simulink model "Cruise_Model_RebuildControl"  (R2024a)
settings: Solver=ode23t  StartTime=0.0  StopTime=20  RelTol=1e-3
values from neighbouring files (symbols this model uses):
  coefficients =     [UAM2.mat]    (also in VX4_cur.mat; VX4data.mat; alexisignoringme11UAM2.mat; alexisignoringme12.mat)
  K = lqr(sys, Q, R)    [QRerr.m]    (also in QRerr_p.m; alexisignoringme4.mat = [-2.3054870934e-16 -3.29424508508e-08 -2.01640092228e-07 -0.; alexisignoringme5.mat = [-2.3054870934e-16 -3.29424508508e-08 -2.01640092228e-07 -0.; alexisignoringme6.mat = [-2.3054870934e-16 -3.29424508508e-08 -2.01640092228e-07 -0.)
  mission =     [alexisignoringme.mat]    (also in alexisignoringme11UAM2.mat; alexisignoringme12.mat; alexisignoringme13.mat; alexisignoringme14.mat)
  q = 0.5*1.225*airflow.U^2    [VLMV3.m]    (also in VLMV3_modified.m = 0.5*1.225*airflow.U^2*Sref)
  referenceGeo =     [VX4data.mat]    (also in alexisignoringme.mat; alexisignoringme11UAM2.mat; alexisignoringme12.mat; alexisignoringme13.mat)
  Ue = U(:,idx(2)+1)    [QRerr.m]    (also in QRerr_LQI.m; QRerr_p.m; alexisignoringme4.mat = [0.01662518914 6.61806403433e-08 9.21309449136e-07 1460.2523; alexisignoringme5.mat = [0 0 0 0 0 -1471.90874183 1.06985703496e-06 -4.11944256484e-)
  X = [0.00351660116596 0 -9.99999602467 0 0 0 2.75026701025e-08 -4.1982332666e-06 -1.5333765693e-08 0.000503097278932 0 -6.54626389426e-11 ... (630 elements, 9x5x14)]    [alexisignoringme.mat]    (also in alexisignoringme12.mat = [0.000256495736971 0 -9.99999647184 0 0 0 0 -3.73764411116e-; alexisignoringme13.mat = [0.00833666803911 0 -10.0000021435 0 0 0 0 7.14203458163e-06; alexisignoringme14.mat = [0.00833666803911 0 -10.0000021435 0 0 0 0 7.14203458163e-06; alexisignoringme4.mat = [0.00351658839646 0 -9.99999599468 0 0 0 2.7327442949e-09 -4)
  Xes = X(:,idx(2))    [QRerr.m]    (also in QRerr_LQI.m; QRerr_p.m; alexisignoringme4.mat = [0.00351658839646 0 -9.99999599468 0 0 0 2.7327442949e-09 -4; alexisignoringme5.mat = [0 0 -1.11199998303 0 0 0 -1.38069247376e-09 1.48137256273e-)
undefined symbols (not defined in the file or in its folder): F, Light, MIL, VX4
libraries: slpidlib x14, aerolibwind2 x8, aerolibatmos2 x4, shared6dof x1
(part 1 of 3)
settings Model: Creator=Jem  LastModifiedBy=Jem
settings OptimizationCC: ReuseModelBlockBuffer=off
settings RTWCC: GPUComputeCapability=3.5

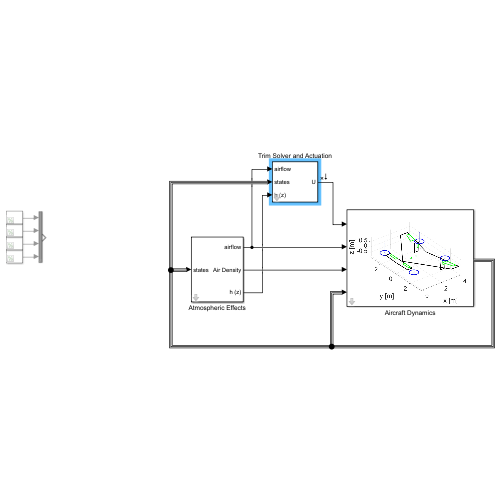
[thumbnail: Simulink's stored preview of the top-level diagram]
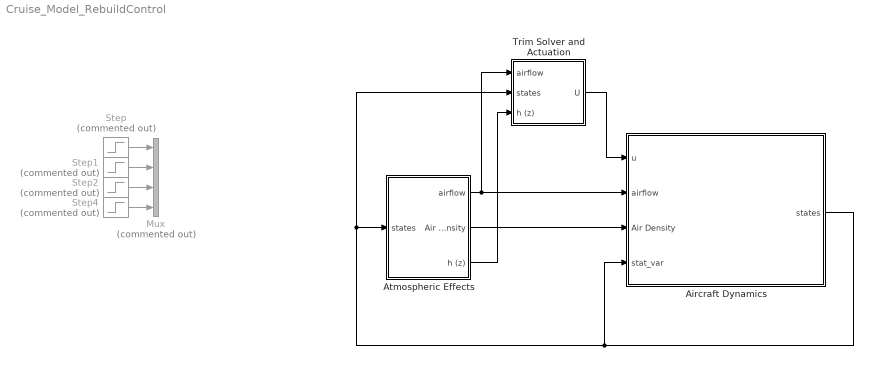
== system Cruise_Model_RebuildControl ==
  Aircraft Dynamics : Subsystem  mask{stabDeriv_local=0, config=VX4, refGeo=VX4.refGeo, mesh=[], stabDeriv=coefficients, I=[107 0 0.6971;0 93 0;0.6971 0 196], ac=[2.04 0 0], cg=[1.51 0 0], m=150, uvw=Xes(1:3), lmn=Xes(7:9), pqr=Xes(4:6), xyz_e=[0 0 0], CD0=0.038, CL0=0.3, Cm0=-0.02, CDa=0.1194, CLa=3.9492, CYa=0, CDb=0, CLb=0, CYb=-0.1997, Clla=0, Cma=-0.3679, Cna=0, Cllb=-0.1796, Cmb=0, Cnb=0.0421, CDn=[0 0 0], CLn=[0.1977 0 0], CYn=[0 0.01532 0.0984], Clln=[0 0.1366 -0.0126], Cmn=[0.2941 0 0], Cnn=[0 -0.0107 -0.03229], CYp=-0.1211, CYr=0.2494, CLq=4.7784, Clp=-0.3291, Clr=0.1134, Cmq=-2.4803, Cnp=0.01634, Cnr=-0.0387, kt=[3.13e-05;3.13e-05;3.13e-05;3.13e-05], kb=[7.5e-07;7.5e-07;7.5e-07;7.5e-07], Tinit=[0 0 0 0], xyz_tr=[3.7 1.75 0;3.7 -1.75 0;0.25 -2 0;0.25 2 0], anginit=[0 0 0;0 0 0;0 0 0;0 0 0], max_def_tr=[1 -1;1 -1;1 -1;1 -1], dir=[1;-1;1;-1]}
      mask prompts: config "Configuration (object)"; refGeo "Reference Geometry (struct)"; mesh "Mesh (struct)"; stabDeriv "Stability Derivatives (struct)"; I "Inertia Tensor"; ac "Aerodynamic Centre [x y z]_ref"; cg "Centre of Gravity [x y z]_ref"; m "Mass [kg]"; uvw "[u, v, w]"; lmn "[roll, pitch, yaw]"; pqr "[p, q, r]"; xyz_e "[Xe, Ye, Ze]"; CDa "CD_a"; CLa "CL_a"; CYa "CY_a"; CDb "CD_b"; CLb "CL_b"; CYb "CY_b"; Clla "Cl_a"; Cma "Cm_a"; Cna "Cn_a"; Cllb "Cl_b"; Cmb "Cm_b"; Cnb "Cn_b"; CDn "CD_n"; CLn "CL_n"; CYn "CY_n"; Clln "Cl_n"; Cmn "Cm_n"; Cnn "Cn_n"; Tinit "Initial Thrust [kN]"; xyz_tr "XYZ_b Pos [m]"; anginit "Initial ang_b [rad]"; max_def_tr "Max [+ve -ve] Deflection (from baseline) [rad]"; dir "Rot. Dir. ([1:Clockwise, -1:Anticlockwise])"
      mask Callback config:
      | config = get_param(gcb, 'config');
      |     m = Simulink.Mask.get(gcb);
      | 
      |     if config ~= "[]"
      |     try
      |         I = evalin('base',[config '.I']);
      |         I_mask = m.getParameter('I');
      |         I_mask.Value = mat2str(I);
      | 
      |         CoL = evalin('base', [config '.CoL']);
      |         CoL_mask = m.getParameter('ac');
      |         CoL_mask.Value = mat2str(CoL);
      | 
      |         CG = evalin('base', [config '.CG']);
      |         CG_mask = m.getParameter('cg');
      |         CG_mask.Value = mat2str(CG);
      | 
      |         Cd0 = evalin('base', [config '.Cd0']);
      |         Cd0_mask = m.getParameter('CD0');
      |         Cd0_mask.Value = mat2str(Cd0);
      | 
      |         mass = evalin('base', [config '.m']);
      |         mass_mask = m.getParameter('m');
      |         mass_mask.Value = mat2str(mass);
      | 
      |         thrustObjs = evalin('base', [config '.thrust']);
      |         xyz_tr = m.getParameter('xyz_tr');
      |         anginit = m.getParameter('anginit');
      |         max_def_tr = m.getParameter('max_def_tr');
      |         Tinit = m.getParameter('Tinit');
      | 
      |         kb = m.getParameter('kb');
      |         kt = m.getParameter('kt');
      |         dir = m.getParameter('dir');
      | 
      |         xyz_tr_temp = zeros(length(thrustObjs.rotors), 3);
      |         anginit_temp = zeros(length(thrustObjs.rotors), 3);
      |         max_def_tr_temp = zeros(length(thrustObjs.rotors), 2);
      | 
      |         kb_temp = zeros(length(thrustObjs.rotors), 1);
      |         kt_temp = zeros(length(thrustObjs.rotors), 1);
      |         dir_temp = zeros(length(thrustObjs.rotors), 1);
      | 
      |         for i = 1:length(thrustObjs.rotors)
      |             xyz_tr_temp(i,1:3) = thrustObjs.rotors(i).pos;
      |             anginit_temp(i,1:3) = thrustObjs.rotors(i).ang;
      |             max_def_tr_temp(i,1:2) = thrustObjs.rotors(i).maxdef;
      | 
      |             kb_temp(i,1) = thrustObjs.rotors(i).kb;
      |             kt_temp(i,1) = thrustObjs.rotors(i).kt;
      |             dir_temp(i,1) = thrustObjs.rotors(i).dir;
      |         end
      | 
      |         xyz_tr.Value = mat2str(xyz_tr_temp);
      |         anginit.Value = mat2str(anginit_temp);
      |         max_def_tr.Value = mat2str(max_def_tr_temp);
      |         Tinit.Value = mat2str(zeros(1, length(thrustObjs.rotors)));
      | 
      |         kb.Value = mat2str(kb_temp);
      |         kt.Value = mat2str(kt_temp);
      |         dir.Value = mat2str(dir_temp);
      | 
      |         Tinit  = get_param(gcb, 'Tinit');
      |         Tinit = str2num(Tinit);
      | 
      |         n = size(Tinit,2); % number of columns
      | 
      |         load('buses.mat', "coeff", "thrust")
      | 
      |         % handled brute forcefully due to comma seperated list
      |         [thrust.Elements.Dimensions] = deal([1,n], [n,3], [n,3], [n,2], [n,1], [n,1], [n,1]);
      | 
      |         save('buses.mat', "coeff", "thrust")
      | 
      |         disp("Configuration data extracted.")
      | 
      |     catch
      |         config = m.getParameter('config');
      |         config.Value = '[]';
      |         error('Data could not be read from specified configuration object. Please enter data manually.')
      |     end
      | 
      |     try
      |         name = get_param(gcb, 'config');
      |         config = evalin('base', name);
      |         plotConfiguration(config,0)
      | 
      |         disp("Image generated.")
      |     catch
      |         warning('Could not generate configuration image.')
      |     end
      | 
      |     end
      mask Callback stabDeriv:
      | stabDeriv = get_param(gcb, 'stabDeriv');
      |     m = Simulink.Mask.get(gcb);
      | 
      |     if stabDeriv ~= "[]"
      |         try
      |             variables = ["CL0", "Cm0", "CD0", "CLa", "CDa", "CYa", ...
      |                 "Clla", "Cma", "Cna", ...
      |                 "CLb", "CDb", "CYb", "Cllb", "Cmb", "Cnb" ...
      |                 "CDn", "CLn", "CYn", "Clln", "Cmn", "Cnn" ...
      |                 "CYp", "CYr", "CLq", "Clp", "Clr", "Cmq", "Cnp", "Cnr"];
      | 
      |             for i = 1:length(variables)
      |               param = char(variables(i));
      | 
      |               if param == "Clla"
      |                   paramws = 'Cla'; % handle case sensitivity
      |               elseif param == "Cllb"
      |                   paramws = 'Clb';
      |               elseif param == "Clln"
      |                   paramws = 'Cln';
      |               else
      |                   paramws = param;
      |               end
      | 
      |               disp(paramws)
      |               var = evalin('base',[stabDeriv '.' paramws]);
      |               var_mask = m.getParameter(param);
      |               var_mask.Value = mat2str(var);
      |               disp('here')
      |             end
      | 
      |         catch
      |           var = m.getParameter('stabDeriv');
      |           var.Value = '[]';
      |           error('Data could not be read from specified structure. Please enter data manually.')
      |         end
      | 
      |         % Handle bus sizing
      |     end
      mask Callback CLn:
      | CLn = get_param(gcb, 'CLn');
      |     n = length(str2num(CLn));
      | 
      |     load('buses.mat', "coeff", "thrust")
      | 
      |     % handled brute forcefully due to comma seperated list
      |     [coeff.Elements.Dimensions] = deal(1,1,1,1,1,1,1,1,1,1,1,1,1,1,1,n,n,n,n,n,n,1,1,1,1,1,1,1,1);
      | 
      |     save('buses.mat', "coeff", "thrust")
      |     clear coeff thrust
      mask Callback Tinit:
      | Tinit  = get_param(gcb, 'Tinit');
      |     Tinit = str2num(Tinit);
      | 
      |     n = size(Tinit,2); % number of columns
      | 
      |     load('buses.mat', "coeff", "thrust")
      | 
      |     % handled brute forcefully due to comma seperated list
      |     [thrust.Elements.Dimensions] = deal([1,n], [n,3], [n,3], [n,2], [n,1], [n,1], [n,1]);
      | 
      |     save('buses.mat', "coeff", "thrust")
      |     clear coeff thrust
      mask DialogControl ParameterGroupVar Prompt: Input Structures/Objects
      mask DialogControl Container6 Prompt: Geometry
      mask DialogControl Container4 Prompt: Initial Conditions
      mask DialogControl Container5 Prompt: Aerodynamic Derivatives
      mask DialogControl Container7 Prompt: Control Derivatives
      mask DialogControl Container8 Prompt: Coupling Derivatives
      mask DialogControl Container9 Prompt: Thrust Components
      mask Display:
      | try
      |     image('config.jpg');
      | catch
      |     image('drone.png');
      | end
  Atmospheric Effects : Subsystem  mask{a=Off, g=Off, t=Off}
      mask prompts: a "Altitude Effects"; g "Gust"; t "Turbulence"
      mask TypeOptions a: On | Off
      mask Callback a: a = get_param(gcb, 'a')
      mask TypeOptions g: On | Off
      mask TypeOptions t: On | Off
  Mux : Mux  Commented=on
  Step : Step  Commented=on  After=0  SampleTime=0
  Step1 : Step  Commented=on  After=0  SampleTime=0
  Step2 : Step  Commented=on  Time=20  After=0.1  SampleTime=0
  Step4 : Step  Commented=on  Time=30  After=0.1  SampleTime=0
  Trim Solver and Actuation : Subsystem  mask{sel=Standard Trim Solver, mission=mission}
      mask prompts: sel "Optimisation Type"; mission "Profile"
      mask TypeOptions sel: PID_GBDP | PID_GBDP_withThrust | Standard Trim Solver
  wires:
  Aircraft Dynamics/1(states) -> Aircraft Dynamics/4(stat_var), Atmospheric Effects/1(states), Trim Solver and Actuation/2(states)
  Step/1 -> Mux/1
  Atmospheric Effects/1(airflow) -> Aircraft Dynamics/2(airflow), Trim Solver and Actuation/1(airflow)
  Atmospheric Effects/2(Air Density) -> Aircraft Dynamics/3(Air Density)
  Step1/1 -> Mux/2
  Step2/1 -> Mux/3
  Step4/1 -> Mux/4
  Atmospheric Effects/3(h (z)) -> Trim Solver and Actuation/3(h (z))
  Trim Solver and Actuation/1(U) -> Aircraft Dynamics/1(u)

== system Cruise_Model_RebuildControl/Aircraft Dynamics ==
  u : Inport
  airflow : Inport  Port=2
  Air Density : Inport  Port=3
  stat_var : Inport  Port=4
  6DoF : shared6dof/6DOF (Euler Angles)  units=Metric (MKS)  mtype=Fixed  rep=Euler Angles  xme_0=xyz_e  Vm_0=uvw  eul_0=lmn  pm_0=pqr  mass_0=m  mass_e=0.5  mass_f=2.0  inertia=I  inertia_e=eye(3)  inertia_f=2*eye(3)  k_quat=1.0  vre_flag=on  abi_flag=off  aMode=0  xme_statename=''  Vm_statename=''  eul_statename=''  quat_statename=''  pm_statename=''  mass_statename=''
  Aerodynamic Forces and Moments : Subsystem
  Bus Creator : BusCreator  Inputs=8
  states : Outport
  wires:
  Aerodynamic Forces and Moments/2(Mcg) -> 6DoF/2  "Mcg"
  Aerodynamic Forces and Moments/1(Fb) -> 6DoF/1  "Fb"
  Bus Creator/1 -> states/1  "states"
  6DoF/2 -> Bus Creator/2  "Xe"
  6DoF/8 -> Bus Creator/8  "A_bb"
  6DoF/4 -> Bus Creator/4  "DCM"
  6DoF/7 -> Bus Creator/7  "pqr_dot"
  6DoF/1 -> Bus Creator/1  "Ve"
  6DoF/6 -> Bus Creator/6  "pqr"
  6DoF/5 -> Bus Creator/5  "uvw"
  6DoF/3 -> Bus Creator/3  "EA"
  airflow/1 -> Aerodynamic Forces and Moments/2(airflow)
  u/1 -> Aerodynamic Forces and Moments/1(U)
  Air Density/1 -> Aerodynamic Forces and Moments/3(Air Density)
  stat_var/1 -> Aerodynamic Forces and Moments/4(stat_var)

== system Cruise_Model_RebuildControl/Atmospheric Effects ==
  states : Inport
  Airflow : Subsystem
  Atmospheric Effects1 : Subsystem
  airflow : Outport
  Air Density : Outport  Port=2
  h (z) : Outport  Port=3
  wires:
  states/1 -> Atmospheric Effects1/1(States), Airflow/2(states)
  Atmospheric Effects1/1(Vw) -> Airflow/1(Vw)
  Airflow/1(airflow) -> airflow/1
  Atmospheric Effects1/2(Air Density) -> Air Density/1
  Atmospheric Effects1/3(h (z)) -> h (z)/1

== system Cruise_Model_RebuildControl/Trim Solver and Actuation ==
  airflow : Inport
  states : Inport  Port=2
  h (z) : Inport  Port=3
  Controller : Subsystem  Variant=on  VariantControl=Choice  mask{sel=sel, mission=mission}
      mask prompts: sel "selection"
      settings: PortSchema="{\"entries\":[{\"content\":{\"sides\":[{\"content\":{\"connectorIds\":[\"In1\",\"In2\",\"In3\"]},\"type\":\"ConnectorPlacement.EquallySpacedRectSide\",\"uuid\":\"c80bf499-6c9e-4c3b-bb20-23bbf7a6035e\"},{\"content\":{\"connectorIds\":[\"Out1\"],\"side\":\"RIGHT\"},\"type\":\"ConnectorPlacement.EquallySpacedRectSide\",\"uuid\":\"d1b7f6ea-e78e-47b9-8a92-dc280984d9ed\"},{\"content\":{\"connectorIds\":[],\"side\":\"TOP\"},\"type\":\"ConnectorPlacement.EquallySpacedRectSide\",\"uuid\":\"c4b261b2-9ac3-4d4e-b6f4-b8885cdc53c4\"},{\"content\":{\"connectorIds\":[\"In4\"],\"side\":\"BOTTOM\"},\"type\":\"ConnectorPlacement.EquallySpacedRectSide\",\"uuid\":\"beb66ba2-4a64-4299-ad5c-3d2a3893b930\"}]},\"type\":\"ConnectorPlacement.EquallySpacedConnector\",\"uuid\":\"9854a30a-2130-48e0-933d-0fb0bd9720d5\"}],\"packageUris\":[\"http://schema.mathworks.com/mf0/Connector/R2020b\"],\"version\":\"1.0\"}"
  Demux : Demux  Outputs=3
  Scope : Scope
  U : Outport
  wires:
  airflow/1 -> Demux/1
  states/1 -> Controller/1(states)
  Demux/1 -> Scope/1, Controller/2(alpha)
  Demux/3 -> Controller/3(Va)
  h (z)/1 -> Controller/4(h (z))
  Controller/1(U) -> U/1

== system Cruise_Model_RebuildControl/Aircraft Dynamics/Aerodynamic Forces and Moments ==
  U : Inport
  airflow : Inport  Port=2
  Air Density : Inport  Port=3
  stat_var : Inport  Port=4
  Bus Selector : BusSelector  OutputSignals=uvw,pqr,EA
  Demux : Demux  Outputs=3
  Gather Thrust Properties : Subsystem
  Gather derivatives : Subsystem
  MATLAB Function : MATLAB Function  InitFcn=load buses.mat  StartFcn=load buses.mat  TreatAsAtomicUnit=on  VariantControl=Choice  mask{refGeo=referenceGeo}
      settings: OpenFcn=load buses.mat
  Mux : Mux  Inputs=3
  Fb : Outport
  Mcg : Outport  Port=2
  wires:
  Demux/3 -> MATLAB Function/5(V)  "V"
  airflow/1 -> Demux/1
  stat_var/1 -> Bus Selector/1
  Bus Selector/1 -> Mux/1  "<uvw>"
  Bus Selector/2 -> Mux/2  "<pqr>"
  Bus Selector/3 -> Mux/3  "<EA>"
  Gather derivatives/1(Out1) -> MATLAB Function/1(coeff)
  U/1 -> MATLAB Function/2(u)
  Demux/1 -> MATLAB Function/3(alpha)
  Demux/2 -> MATLAB Function/4(beta)
  Air Density/1 -> MATLAB Function/6(rho)
  Mux/1 -> MATLAB Function/7(X)
  Gather Thrust Properties/1(Out1) -> MATLAB Function/8(thrust)
  MATLAB Function/1(Fb) -> Fb/1  "fb"
  MATLAB Function/2(Mcg) -> Mcg/1

== system Cruise_Model_RebuildControl/Atmospheric Effects/Airflow ==
  Vw : Inport
  states : Inport  Port=2
  Bus Selector2 : BusSelector  OutputSignals=uvw
  Mux : Mux  Inputs=3
  Subsystem : Subsystem
  airflow : Outport
  wires:
  Mux/1 -> airflow/1
  Vw/1 -> Subsystem/1(Vw)
  Subsystem/3(Va) -> Mux/3
  states/1 -> Bus Selector2/1
  Bus Selector2/1 -> Subsystem/2(uvw)  "<uvw>"
  Subsystem/1(alpha) -> Mux/1
  Subsystem/2(beta) -> Mux/2

== system Cruise_Model_RebuildControl/Atmospheric Effects/Atmospheric Effects1 ==
  States : Inport
  Bus Selection : Subsystem
  Variant Subsystem : Subsystem  Variant=on  mask{a=a, g=g, t=t}
  Vw : Outport
  Air Density : Outport  Port=2
  h (z) : Outport  Port=3
  wires:
  Variant Subsystem/2(Air Density) -> Air Density/1
  States/1 -> Bus Selection/1(States)
  Variant Subsystem/1(Vw) -> Vw/1
  Bus Selection/1(<Ve>) -> Variant Subsystem/1(uvw_e)
  Bus Selection/2(<DCM>) -> Variant Subsystem/2(DCM)
  Bus Selection/3(h (z)) -> h (z)/1, Variant Subsystem/3(h (z))

== system Cruise_Model_RebuildControl/Trim Solver and Actuation/Controller ==
  states : Inport
  alpha : Inport  Port=2
  Va : Inport  Port=3
  h (z) : Inport  Port=4
  PID_GBDP : Subsystem  VariantControl=sel == 1
      settings: PortSchema="{\"entries\":[{\"content\":{\"sides\":[{\"content\":{\"connectorIds\":[\"In1\",\"In2\",\"In3\"]},\"type\":\"ConnectorPlacement.EquallySpacedRectSide\",\"uuid\":\"c80bf499-6c9e-4c3b-bb20-23bbf7a6035e\"},{\"content\":{\"connectorIds\":[\"Out1\"],\"side\":\"RIGHT\"},\"type\":\"ConnectorPlacement.EquallySpacedRectSide\",\"uuid\":\"d1b7f6ea-e78e-47b9-8a92-dc280984d9ed\"},{\"content\":{\"connectorIds\":[],\"side\":\"TOP\"},\"type\":\"ConnectorPlacement.EquallySpacedRectSide\",\"uuid\":\"c4b261b2-9ac3-4d4e-b6f4-b8885cdc53c4\"},{\"content\":{\"connectorIds\":[\"In4\"],\"side\":\"BOTTOM\"},\"type\":\"ConnectorPlacement.EquallySpacedRectSide\",\"uuid\":\"beb66ba2-4a64-4299-ad5c-3d2a3893b930\"}]},\"type\":\"ConnectorPlacement.EquallySpacedConnector\",\"uuid\":\"9854a30a-2130-48e0-933d-0fb0bd9720d5\"}],\"packageUris\":[\"http://schema.mathworks.com/mf0/Connector/R2020b\"],\"version\":\"1.0\"}"
  PID_GBDP_withThrust : Subsystem  VariantControl=sel == 2
  Trim Solver : Subsystem  VariantControl=sel == 3
      settings: PortSchema="{\"entries\":[{\"content\":{\"sides\":[{\"content\":{\"connectorIds\":[\"In1\",\"In2\",\"In3\"]},\"type\":\"ConnectorPlacement.EquallySpacedRectSide\",\"uuid\":\"c80bf499-6c9e-4c3b-bb20-23bbf7a6035e\"},{\"content\":{\"connectorIds\":[\"Out1\"],\"side\":\"RIGHT\"},\"type\":\"ConnectorPlacement.EquallySpacedRectSide\",\"uuid\":\"d1b7f6ea-e78e-47b9-8a92-dc280984d9ed\"},{\"content\":{\"side\":\"TOP\"},\"type\":\"ConnectorPlacement.EquallySpacedRectSide\",\"uuid\":\"c4b261b2-9ac3-4d4e-b6f4-b8885cdc53c4\"},{\"content\":{\"connectorIds\":[\"In4\"],\"side\":\"BOTTOM\"},\"type\":\"ConnectorPlacement.EquallySpacedRectSide\",\"uuid\":\"beb66ba2-4a64-4299-ad5c-3d2a3893b930\"}]},\"type\":\"ConnectorPlacement.EquallySpacedConnector\",\"uuid\":\"9854a30a-2130-48e0-933d-0fb0bd9720d5\"}],\"packageUris\":[\"http://schema.mathworks.com/mf0/Connector/R2020b\"],\"version\":\"1.0\"}"
  U : Outport

== system Cruise_Model_RebuildControl/Aircraft Dynamics/Aerodynamic Forces and Moments/Gather Thrust Properties ==
  note: This subsystem just creates a structure out of the inputs for better handling in the function
  note: i swear there is no better option ):
  Constant : Constant  Value=Tinit
  Constant1 : Constant  Value=xyz_tr
  Constant2 : Constant  Value=anginit
  Constant3 : Constant  Value=max_def_tr
  Constant4 : Constant  Value=kb
  Constant5 : Constant  Value=kt
  Constant6 : Constant  Value=dir
  thrust : BusCreator  Inputs=7  OutDataTypeStr=Bus: thrust
  Out1 : Outport
  wires:
  thrust/1 -> Out1/1  "thrust"
  Constant/1 -> thrust/1  "Tinit"
  Constant1/1 -> thrust/2  "xyz_tr"
  Constant2/1 -> thrust/3  "anginit"
  Constant3/1 -> thrust/4  "max_def_tr"
  Constant4/1 -> thrust/5  "kb"
  Constant5/1 -> thrust/6  "kt"
  Constant6/1 -> thrust/7  "dir"

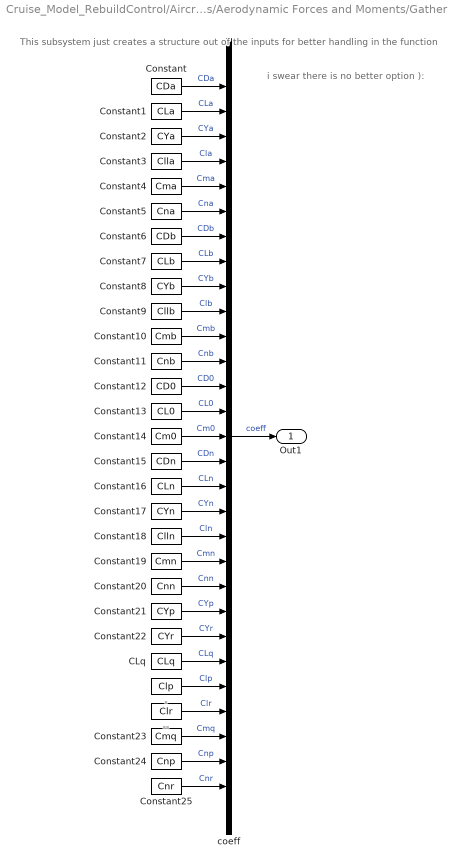
== system Cruise_Model_RebuildControl/Aircraft Dynamics/Aerodynamic Forces and Moments/Gather derivatives ==
  note: i swear there is no better option ):
  note: This subsystem just creates a structure out of the inputs for better handling in the function
  - : Constant  Value=Clp
  -- : Constant  Value=Clr
  CLq : Constant  Value=CLq
  Constant : Constant  Value=CDa
  Constant1 : Constant  Value=CLa
  Constant10 : Constant  Value=Cmb
  Constant11 : Constant  Value=Cnb  VectorParams1D=off
  Constant12 : Constant  Value=CD0
  Constant13 : Constant  Value=CL0
  Constant14 : Constant  Value=Cm0
  Constant15 : Constant  Value=CDn
  Constant16 : Constant  Value=CLn
  Constant17 : Constant  Value=CYn
  Constant18 : Constant  Value=Clln
  Constant19 : Constant  Value=Cmn
  Constant2 : Constant  Value=CYa
  Constant20 : Constant  Value=Cnn
  Constant21 : Constant  Value=CYp
  Constant22 : Constant  Value=CYr
  Constant23 : Constant  Value=Cmq
  Constant24 : Constant  Value=Cnp
  Constant25 : Constant  Value=Cnr
  Constant3 : Constant  Value=Clla
  Constant4 : Constant  Value=Cma
  Constant5 : Constant  Value=Cna
  Constant6 : Constant  Value=CDb
  Constant7 : Constant  Value=CLb
  Constant8 : Constant  Value=CYb
  Constant9 : Constant  Value=Cllb
  coeff : BusCreator  Inputs=29
  Out1 : Outport
  wires:
  coeff/1 -> Out1/1  "coeff"
  Constant/1 -> coeff/1  "CDa"
  Constant1/1 -> coeff/2  "CLa"
  Constant2/1 -> coeff/3  "CYa"
  Constant3/1 -> coeff/4  "Cla"
  Constant4/1 -> coeff/5  "Cma"
  Constant5/1 -> coeff/6  "Cna"
  Constant11/1 -> coeff/12  "Cnb"
  Constant10/1 -> coeff/11  "Cmb"
  Constant9/1 -> coeff/10  "Clb"
  Constant8/1 -> coeff/9  "CYb"
  Constant7/1 -> coeff/8  "CLb"
  Constant6/1 -> coeff/7  "CDb"
  Constant12/1 -> coeff/13  "CD0"
  Constant13/1 -> coeff/14  "CL0"
  Constant14/1 -> coeff/15  "Cm0"
  Constant15/1 -> coeff/16  "CDn"
  Constant16/1 -> coeff/17  "CLn"
  Constant17/1 -> coeff/18  "CYn"
  Constant18/1 -> coeff/19  "Cln"
  Constant19/1 -> coeff/20  "Cmn"
  Constant20/1 -> coeff/21  "Cnn"
  Constant21/1 -> coeff/22  "CYp"
  Constant22/1 -> coeff/23  "CYr"
  CLq/1 -> coeff/24  "CLq"
  -/1 -> coeff/25  "Clp"
  --/1 -> coeff/26  "Clr"
  Constant23/1 -> coeff/27  "Cmq"
  Constant24/1 -> coeff/28  "Cnp"
  Constant25/1 -> coeff/29  "Cnr"

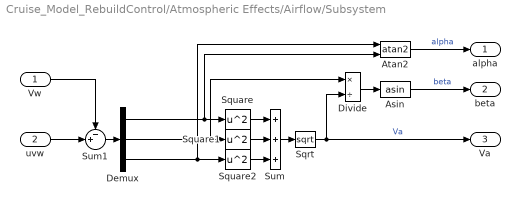
== system Cruise_Model_RebuildControl/Atmospheric Effects/Airflow/Subsystem ==
  Vw : Inport
  uvw : Inport  Port=2
  Asin : Trigonometry  Operator=asin
  Atan2 : Trigonometry  Operator=atan2
  Demux : Demux  Outputs=3
  Divide : Product  Inputs=*/
  Sqrt : Sqrt
  Square : Math  Operator=square
  Square1 : Math  Operator=square
  Square2 : Math  Operator=square
  Sum : Sum  Inputs=+++
  Sum1 : Sum  Inputs=-+|
  alpha : Outport
  beta : Outport  Port=2
  Va : Outport  Port=3
  wires:
  Asin/1 -> beta/1  "beta"
  Atan2/1 -> alpha/1  "alpha"
  Vw/1 -> Sum1/1
  uvw/1 -> Sum1/2
  Sum/1 -> Sqrt/1
  Divide/1 -> Asin/1
  Sqrt/1 -> Divide/2, Va/1  "Va"
  Square1/1 -> Sum/2
  Square/1 -> Sum/1
  Demux/1 -> Atan2/2, Square/1
  Demux/2 -> Square1/1, Divide/1
  Sum1/1 -> Demux/1
  Square2/1 -> Sum/3
  Demux/3 -> Atan2/1, Square2/1

== system Cruise_Model_RebuildControl/Atmospheric Effects/Atmospheric Effects1/Bus Selection ==
  States : Inport
  Bus Selector1 : BusSelector  OutputSignals=Xe
  Demux : Demux  Outputs=3
  r : BusSelector  OutputSignals=Ve,DCM
  <Ve> : Outport
  <DCM> : Outport  Port=2
  h (z) : Outport  Port=3
  wires:
  r/2 -> <DCM>/1  "<DCM>"
  States/1 -> Bus Selector1/1, r/1
  Bus Selector1/1 -> Demux/1  "<Xe>"
  Demux/3 -> h (z)/1  "h (x)"
  r/1 -> <Ve>/1  "<Ve>"

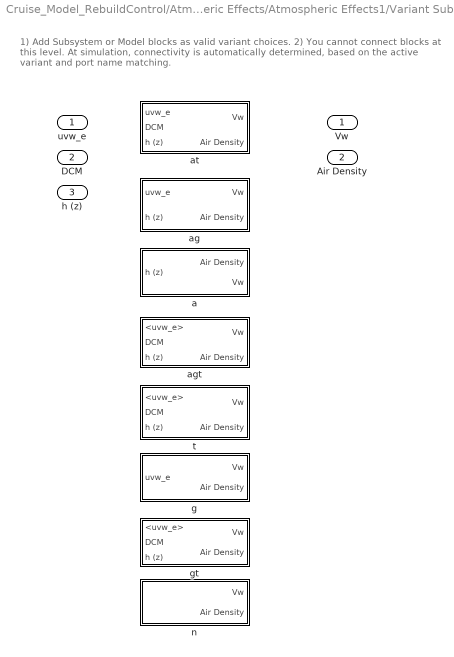
== system Cruise_Model_RebuildControl/Atmospheric Effects/Atmospheric Effects1/Variant Subsystem ==
  note: 1) Add Subsystem or Model blocks as valid variant choices.
      | 2) You cannot connect blocks at this level. At simulation, connectivity is automatically
      | determined, based on the active variant and port name matching.
  uvw_e : Inport
  DCM : Inport  Port=2
  h (z) : Inport  Port=3
  a : Subsystem  VariantControl=a == 1 && g ~= 1 && t ~= 1
  ag : Subsystem  VariantControl=a == 1 && g == 1 && t ~= 1
  agt : Subsystem  VariantControl=a == 1 && g == 1 && t == 1
  at : Subsystem  VariantControl=a == 1 && g ~= 1 && t == 1
  g : Subsystem  VariantControl=a ~= 1 && g == 1 && t ~= 1
  gt : Subsystem  VariantControl=a ~= 1 && g == 1 && t == 1
  n : Subsystem  VariantControl=a ~= 1 && g ~= 1 && t ~= 1
  t : Subsystem  VariantControl=a ~= 1 && g ~= 1 && t == 1
  Vw : Outport
  Air Density : Outport  Port=2

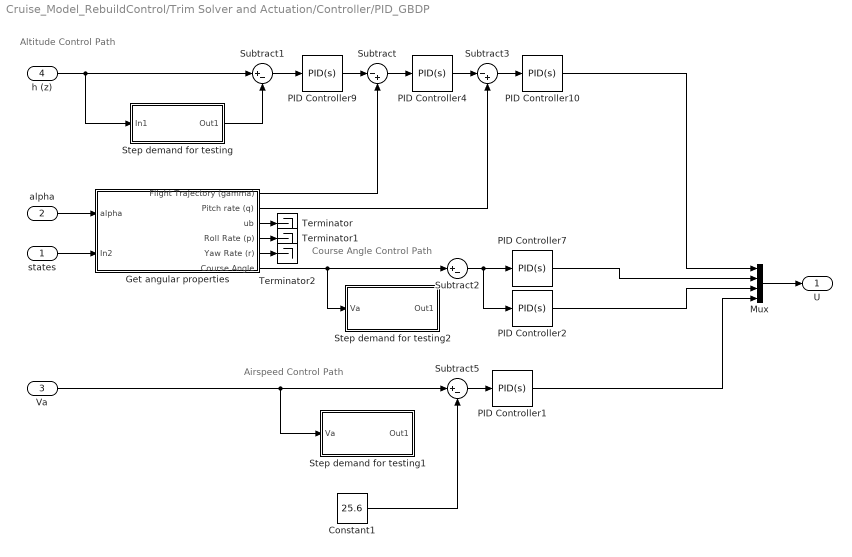
== system Cruise_Model_RebuildControl/Trim Solver and Actuation/Controller/PID_GBDP ==
  note: Altitude Control Path
  note: Airspeed Control Path
  note: Course Angle Control Path
  states : Inport
  alpha : Inport  Port=2
  Va : Inport  Port=3
  h (z) : Inport  Port=4
  Constant1 : Constant  Value=25.6
  Get angular properties : Subsystem
  Mux : Mux
  PID Controller1 : slpidlib/PID Controller  Controller=PID  Form=Parallel  TimeDomain=Continuous-time  UseExternalTs=off  SampleTime=-1  IntegratorMethod=Forward Euler  FilterMethod=Forward Euler  ControllerParametersSource=internal  P=-124.171962714531  I=-8.86566238209981  UseKiTs=off  D=35.5117343437496  UseExternalDerivativeSource=off  N=0.73276571825447  UseFilter=on  TunerSelectOption=Transfer Function Based (PID Tuner App)  InitialConditionSource=internal  InitialConditionForIntegrator=0  InitialConditionForFilter=1  DifferentiatorICPrevScaledInput=0  ExternalReset=none  TrackingMode=off  Kt=1  LimitOutput=on  SatLimitsSource=internal  UpperSaturationLimit=300  LowerSaturationLimit=0  LinearizeAsGain=on  AntiWindupMode=clamping  Kb=1  LimitIntegrator=off  UpperIntegratorSaturationLimit=inf  LowerIntegratorSaturationLimit=-inf  POutMin=[]  POutMax=[]  IOutMin=[]  IOutMax=[]  DOutMin=[]  DOutMax=[]  NOutMin=[]  NOutMax=[]  SumOutMin=[]  SumOutMax=[]  SaturationOutMin=[]  SaturationOutMax=[]  PParamMin=[]  PParamMax=[]  IParamMin=[]  IParamMax=[]  DParamMin=[]  DParamMax=[]  NParamMin=[]  NParamMax=[]  KbParamMin=[]  KbParamMax=[]  KtParamMin=[]  KtParamMax=[]  KbOutMin=[]  KbOutMax=[]  KtOutMin=[]  KtOutMax=[]  IntegratorOutMin=[]  IntegratorOutMax=[]  FilterOutMin=[]  FilterOutMax=[]  SumI1OutMin=[]  SumI1OutMax=[]  SumI2OutMin=[]  SumI2OutMax=[]  SumI3OutMin=[]  SumI3OutMax=[]  SumI4OutMin=[]  SumI4OutMax=[]  SumDOutMin=[]  SumDOutMax=[]  DifferentiatorOutMin=[]  DifferentiatorOutMax=[]  FilterDiffOutCoefMin=[]  FilterDiffOutCoefMax=[]  ReciprocalOutMin=[]  ReciprocalOutMax=[]  SumDenOutMin=[]  SumDenOutMax=[]  SumNumOutMin=[]  SumNumOutMax=[]  DivideOutMin=[]  DivideOutMax=[]  UdiffTsProdOutMin=[]  UdiffTsProdOutMax=[]  NTsProdOutMin=[]  NTsProdOutMax=[]  UintegralTsProdOutMin=[]  UintegralTsProdOutMax=[]  UngainTsProdOutMin=[]  UngainTsProdOutMax=[]  ClampingZeroOutDataTypeStr=Inherit: Inherit via back propagation  ClampingZeroOutMin=[]  ClampingZeroOutMax=[]  FilterDenConstantOutDataTypeStr=Inherit: Inherit via back propagation  FilterDenConstantOutMin=[]  FilterDenConstantOutMax=[]  PCopyOutDataTypeStr=Inherit: Inherit via back propagation  PCopyOutMin=[]  PCopyOutMax=[]  NCopyOutDataTypeStr=Inherit: Inherit via back propagation  NCopyOutMin=[]  NCopyOutMax=[]  IntegratorContinuousStateAttributes=''  IntegratorStateMustResolveToSignalObject=off  IntegratorRTWStateStorageClass=Auto  FilterContinuousStateAttributes=''  FilterStateMustResolveToSignalObject=off  FilterRTWStateStorageClass=Auto  ParallelPVariant=InternalParameters  IdealPVariant=Disabled  IVariant=InternalParameters  DVariant=InternalParameters  IntegratorVariant=Continuous  SatVariant=Enabled  AWVariant=ContClampingParallel  PCopyVariant=Disabled  TRVariant=Disabled  FdbkBlocksVariant=Forward  IdealPFdbkVariant=Disabled  SatFdbkVariant=Disabled  DerivativeFilterVariant=ContFilter  NVariant=InternalParameters  NCopyVariant=Disabled  FilterICVariant=InternalICsFilter  IntegratorICVariant=InternalICs  ExternalResetVariant=Disabled  TRSumVariant=Passthrough  SumFdbkVariant=Disabled  SumVariant=Sum_PID  TsampFilterVariant=InternalTs  TsampNgainVariant=Passthrough  TsampIntegralVariant=Disabled_SignalSpec  ExternalSaturationOutDataTypeStr=Inherit: Same as second input  DerivativeSourceVariant=ErrorSignal
  PID Controller10 : slpidlib/PID Controller  Controller=PID  Form=Parallel  TimeDomain=Continuous-time  UseExternalTs=off  SampleTime=-1  IntegratorMethod=Forward Euler  FilterMethod=Forward Euler  ControllerParametersSource=internal  P=-0.89713711901533  I=-27.659938076894  UseKiTs=off  D=-0.00302643608728309  UseExternalDerivativeSource=off  N=142.832860389355  UseFilter=on  TunerSelectOption=Transfer Function Based (PID Tuner App)  InitialConditionSource=internal  InitialConditionForIntegrator=0.44  InitialConditionForFilter=0  DifferentiatorICPrevScaledInput=0  ExternalReset=none  TrackingMode=off  Kt=1  LimitOutput=on  SatLimitsSource=internal  UpperSaturationLimit=0.44  LowerSaturationLimit=-0.44  LinearizeAsGain=on  AntiWindupMode=clamping  Kb=1  LimitIntegrator=off  UpperIntegratorSaturationLimit=inf  LowerIntegratorSaturationLimit=-inf  POutMin=[]  POutMax=[]  IOutMin=[]  IOutMax=[]  DOutMin=[]  DOutMax=[]  NOutMin=[]  NOutMax=[]  SumOutMin=[]  SumOutMax=[]  SaturationOutMin=[]  SaturationOutMax=[]  PParamMin=[]  PParamMax=[]  IParamMin=[]  IParamMax=[]  DParamMin=[]  DParamMax=[]  NParamMin=[]  NParamMax=[]  KbParamMin=[]  KbParamMax=[]  KtParamMin=[]  KtParamMax=[]  KbOutMin=[]  KbOutMax=[]  KtOutMin=[]  KtOutMax=[]  IntegratorOutMin=[]  IntegratorOutMax=[]  FilterOutMin=[]  FilterOutMax=[]  SumI1OutMin=[]  SumI1OutMax=[]  SumI2OutMin=[]  SumI2OutMax=[]  SumI3OutMin=[]  SumI3OutMax=[]  SumI4OutMin=[]  SumI4OutMax=[]  SumDOutMin=[]  SumDOutMax=[]  DifferentiatorOutMin=[]  DifferentiatorOutMax=[]  FilterDiffOutCoefMin=[]  FilterDiffOutCoefMax=[]  ReciprocalOutMin=[]  ReciprocalOutMax=[]  SumDenOutMin=[]  SumDenOutMax=[]  SumNumOutMin=[]  SumNumOutMax=[]  DivideOutMin=[]  DivideOutMax=[]  UdiffTsProdOutMin=[]  UdiffTsProdOutMax=[]  NTsProdOutMin=[]  NTsProdOutMax=[]  UintegralTsProdOutMin=[]  UintegralTsProdOutMax=[]  UngainTsProdOutMin=[]  UngainTsProdOutMax=[]  ClampingZeroOutDataTypeStr=Inherit: Inherit via back propagation  ClampingZeroOutMin=[]  ClampingZeroOutMax=[]  FilterDenConstantOutDataTypeStr=Inherit: Inherit via back propagation  FilterDenConstantOutMin=[]  FilterDenConstantOutMax=[]  PCopyOutDataTypeStr=Inherit: Inherit via back propagation  PCopyOutMin=[]  PCopyOutMax=[]  NCopyOutDataTypeStr=Inherit: Inherit via back propagation  NCopyOutMin=[]  NCopyOutMax=[]  IntegratorContinuousStateAttributes=''  IntegratorStateMustResolveToSignalObject=off  IntegratorRTWStateStorageClass=Auto  FilterContinuousStateAttributes=''  FilterStateMustResolveToSignalObject=off  FilterRTWStateStorageClass=Auto  ParallelPVariant=InternalParameters  IdealPVariant=Disabled  IVariant=InternalParameters  DVariant=InternalParameters  IntegratorVariant=Continuous  SatVariant=Enabled  AWVariant=ContClampingParallel  PCopyVariant=Disabled  TRVariant=Disabled  FdbkBlocksVariant=Forward  IdealPFdbkVariant=Disabled  SatFdbkVariant=Disabled  DerivativeFilterVariant=ContFilter  NVariant=InternalParameters  NCopyVariant=Disabled  FilterICVariant=InternalICsFilter  IntegratorICVariant=InternalICs  ExternalResetVariant=Disabled  TRSumVariant=Passthrough  SumFdbkVariant=Disabled  SumVariant=Sum_PID  TsampFilterVariant=InternalTs  TsampNgainVariant=Passthrough  TsampIntegralVariant=Disabled_SignalSpec  ExternalSaturationOutDataTypeStr=Inherit: Same as second input  DerivativeSourceVariant=ErrorSignal
  PID Controller2 : slpidlib/PID Controller  Controller=PID  Form=Parallel  TimeDomain=Continuous-time  UseExternalTs=off  SampleTime=-1  IntegratorMethod=Forward Euler  FilterMethod=Forward Euler  ControllerParametersSource=internal  P=0.61259661356046  I=0.000997427544306601  UseKiTs=off  D=0.894500555152138  UseExternalDerivativeSource=off  N=62.5354170285902  UseFilter=on  TunerSelectOption=Transfer Function Based (PID Tuner App)  InitialConditionSource=internal  InitialConditionForIntegrator=0  InitialConditionForFilter=0  DifferentiatorICPrevScaledInput=0  ExternalReset=none  TrackingMode=off  Kt=1  LimitOutput=on  SatLimitsSource=internal  UpperSaturationLimit=0.52  LowerSaturationLimit=-0.52  LinearizeAsGain=on  AntiWindupMode=clamping  Kb=1  LimitIntegrator=off  UpperIntegratorSaturationLimit=inf  LowerIntegratorSaturationLimit=-inf  POutMin=[]  POutMax=[]  IOutMin=[]  IOutMax=[]  DOutMin=[]  DOutMax=[]  NOutMin=[]  NOutMax=[]  SumOutMin=[]  SumOutMax=[]  SaturationOutMin=[]  SaturationOutMax=[]  PParamMin=[]  PParamMax=[]  IParamMin=[]  IParamMax=[]  DParamMin=[]  DParamMax=[]  NParamMin=[]  NParamMax=[]  KbParamMin=[]  KbParamMax=[]  KtParamMin=[]  KtParamMax=[]  KbOutMin=[]  KbOutMax=[]  KtOutMin=[]  KtOutMax=[]  IntegratorOutMin=[]  IntegratorOutMax=[]  FilterOutMin=[]  FilterOutMax=[]  SumI1OutMin=[]  SumI1OutMax=[]  SumI2OutMin=[]  SumI2OutMax=[]  SumI3OutMin=[]  SumI3OutMax=[]  SumI4OutMin=[]  SumI4OutMax=[]  SumDOutMin=[]  SumDOutMax=[]  DifferentiatorOutMin=[]  DifferentiatorOutMax=[]  FilterDiffOutCoefMin=[]  FilterDiffOutCoefMax=[]  ReciprocalOutMin=[]  ReciprocalOutMax=[]  SumDenOutMin=[]  SumDenOutMax=[]  SumNumOutMin=[]  SumNumOutMax=[]  DivideOutMin=[]  DivideOutMax=[]  UdiffTsProdOutMin=[]  UdiffTsProdOutMax=[]  NTsProdOutMin=[]  NTsProdOutMax=[]  UintegralTsProdOutMin=[]  UintegralTsProdOutMax=[]  UngainTsProdOutMin=[]  UngainTsProdOutMax=[]  ClampingZeroOutDataTypeStr=Inherit: Inherit via back propagation  ClampingZeroOutMin=[]  ClampingZeroOutMax=[]  FilterDenConstantOutDataTypeStr=Inherit: Inherit via back propagation  FilterDenConstantOutMin=[]  FilterDenConstantOutMax=[]  PCopyOutDataTypeStr=Inherit: Inherit via back propagation  PCopyOutMin=[]  PCopyOutMax=[]  NCopyOutDataTypeStr=Inherit: Inherit via back propagation  NCopyOutMin=[]  NCopyOutMax=[]  IntegratorContinuousStateAttributes=''  IntegratorStateMustResolveToSignalObject=off  IntegratorRTWStateStorageClass=Auto  FilterContinuousStateAttributes=''  FilterStateMustResolveToSignalObject=off  FilterRTWStateStorageClass=Auto  ParallelPVariant=InternalParameters  IdealPVariant=Disabled  IVariant=InternalParameters  DVariant=InternalParameters  IntegratorVariant=Continuous  SatVariant=Enabled  AWVariant=ContClampingParallel  PCopyVariant=Disabled  TRVariant=Disabled  FdbkBlocksVariant=Forward  IdealPFdbkVariant=Disabled  SatFdbkVariant=Disabled  DerivativeFilterVariant=ContFilter  NVariant=InternalParameters  NCopyVariant=Disabled  FilterICVariant=InternalICsFilter  IntegratorICVariant=InternalICs  ExternalResetVariant=Disabled  TRSumVariant=Passthrough  SumFdbkVariant=Disabled  SumVariant=Sum_PID  TsampFilterVariant=InternalTs  TsampNgainVariant=Passthrough  TsampIntegralVariant=Disabled_SignalSpec  ExternalSaturationOutDataTypeStr=Inherit: Same as second input  DerivativeSourceVariant=ErrorSignal
  PID Controller4 : slpidlib/PID Controller  Controller=PID  Form=Parallel  TimeDomain=Continuous-time  UseExternalTs=off  SampleTime=-1  IntegratorMethod=Forward Euler  FilterMethod=Forward Euler  ControllerParametersSource=internal  P=-0.487630187489664  I=-0.0704619791070383  UseKiTs=off  D=-0.813392530162756  UseExternalDerivativeSource=off  N=7.99704030727873  UseFilter=on  TunerSelectOption=Transfer Function Based (PID Tuner App)  InitialConditionSource=internal  InitialConditionForIntegrator=0.1  InitialConditionForFilter=0  DifferentiatorICPrevScaledInput=0  ExternalReset=none  TrackingMode=off  Kt=1  LimitOutput=on  SatLimitsSource=internal  UpperSaturationLimit=0.44  LowerSaturationLimit=-0.44  LinearizeAsGain=on  AntiWindupMode=clamping  Kb=1  LimitIntegrator=off  UpperIntegratorSaturationLimit=inf  LowerIntegratorSaturationLimit=-inf  POutMin=[]  POutMax=[]  IOutMin=[]  IOutMax=[]  DOutMin=[]  DOutMax=[]  NOutMin=[]  NOutMax=[]  SumOutMin=[]  SumOutMax=[]  SaturationOutMin=[]  SaturationOutMax=[]  PParamMin=[]  PParamMax=[]  IParamMin=[]  IParamMax=[]  DParamMin=[]  DParamMax=[]  NParamMin=[]  NParamMax=[]  KbParamMin=[]  KbParamMax=[]  KtParamMin=[]  KtParamMax=[]  KbOutMin=[]  KbOutMax=[]  KtOutMin=[]  KtOutMax=[]  IntegratorOutMin=[]  IntegratorOutMax=[]  FilterOutMin=[]  FilterOutMax=[]  SumI1OutMin=[]  SumI1OutMax=[]  SumI2OutMin=[]  SumI2OutMax=[]  SumI3OutMin=[]  SumI3OutMax=[]  SumI4OutMin=[]  SumI4OutMax=[]  SumDOutMin=[]  SumDOutMax=[]  DifferentiatorOutMin=[]  DifferentiatorOutMax=[]  FilterDiffOutCoefMin=[]  FilterDiffOutCoefMax=[]  ReciprocalOutMin=[]  ReciprocalOutMax=[]  SumDenOutMin=[]  SumDenOutMax=[]  SumNumOutMin=[]  SumNumOutMax=[]  DivideOutMin=[]  DivideOutMax=[]  UdiffTsProdOutMin=[]  UdiffTsProdOutMax=[]  NTsProdOutMin=[]  NTsProdOutMax=[]  UintegralTsProdOutMin=[]  UintegralTsProdOutMax=[]  UngainTsProdOutMin=[]  UngainTsProdOutMax=[]  ClampingZeroOutDataTypeStr=Inherit: Inherit via back propagation  ClampingZeroOutMin=[]  ClampingZeroOutMax=[]  FilterDenConstantOutDataTypeStr=Inherit: Inherit via back propagation  FilterDenConstantOutMin=[]  FilterDenConstantOutMax=[]  PCopyOutDataTypeStr=Inherit: Inherit via back propagation  PCopyOutMin=[]  PCopyOutMax=[]  NCopyOutDataTypeStr=Inherit: Inherit via back propagation  NCopyOutMin=[]  NCopyOutMax=[]  IntegratorContinuousStateAttributes=''  IntegratorStateMustResolveToSignalObject=off  IntegratorRTWStateStorageClass=Auto  FilterContinuousStateAttributes=''  FilterStateMustResolveToSignalObject=off  FilterRTWStateStorageClass=Auto  ParallelPVariant=InternalParameters  IdealPVariant=Disabled  IVariant=InternalParameters  DVariant=InternalParameters  IntegratorVariant=Continuous  SatVariant=Enabled  AWVariant=ContClampingParallel  PCopyVariant=Disabled  TRVariant=Disabled  FdbkBlocksVariant=Forward  IdealPFdbkVariant=Disabled  SatFdbkVariant=Disabled  DerivativeFilterVariant=ContFilter  NVariant=InternalParameters  NCopyVariant=Disabled  FilterICVariant=InternalICsFilter  IntegratorICVariant=InternalICs  ExternalResetVariant=Disabled  TRSumVariant=Passthrough  SumFdbkVariant=Disabled  SumVariant=Sum_PID  TsampFilterVariant=InternalTs  TsampNgainVariant=Passthrough  TsampIntegralVariant=Disabled_SignalSpec  ExternalSaturationOutDataTypeStr=Inherit: Same as second input  DerivativeSourceVariant=ErrorSignal
  PID Controller7 : slpidlib/PID Controller  Controller=PID  Form=Parallel  TimeDomain=Continuous-time  UseExternalTs=off  SampleTime=-1  IntegratorMethod=Forward Euler  FilterMethod=Forward Euler  ControllerParametersSource=internal  P=0.013462751880451  I=6.03710934436948e-04  UseKiTs=off  D=0.667051880736134  UseExternalDerivativeSource=off  N=87.8445721553921  UseFilter=on  TunerSelectOption=Transfer Function Based (PID Tuner App)  InitialConditionSource=internal  InitialConditionForIntegrator=0  InitialConditionForFilter=0  DifferentiatorICPrevScaledInput=0  ExternalReset=none  TrackingMode=off  Kt=1  LimitOutput=on  SatLimitsSource=internal  UpperSaturationLimit=0.52  LowerSaturationLimit=-0.52  LinearizeAsGain=on  AntiWindupMode=none  Kb=1  LimitIntegrator=off  UpperIntegratorSaturationLimit=inf  LowerIntegratorSaturationLimit=-inf  POutMin=[]  POutMax=[]  IOutMin=[]  IOutMax=[]  DOutMin=[]  DOutMax=[]  NOutMin=[]  NOutMax=[]  SumOutMin=[]  SumOutMax=[]  SaturationOutMin=[]  SaturationOutMax=[]  PParamMin=[]  PParamMax=[]  IParamMin=[]  IParamMax=[]  DParamMin=[]  DParamMax=[]  NParamMin=[]  NParamMax=[]  KbParamMin=[]  KbParamMax=[]  KtParamMin=[]  KtParamMax=[]  KbOutMin=[]  KbOutMax=[]  KtOutMin=[]  KtOutMax=[]  IntegratorOutMin=[]  IntegratorOutMax=[]  FilterOutMin=[]  FilterOutMax=[]  SumI1OutMin=[]  SumI1OutMax=[]  SumI2OutMin=[]  SumI2OutMax=[]  SumI3OutMin=[]  SumI3OutMax=[]  SumI4OutMin=[]  SumI4OutMax=[]  SumDOutMin=[]  SumDOutMax=[]  DifferentiatorOutMin=[]  DifferentiatorOutMax=[]  FilterDiffOutCoefMin=[]  FilterDiffOutCoefMax=[]  ReciprocalOutMin=[]  ReciprocalOutMax=[]  SumDenOutMin=[]  SumDenOutMax=[]  SumNumOutMin=[]  SumNumOutMax=[]  DivideOutMin=[]  DivideOutMax=[]  UdiffTsProdOutMin=[]  UdiffTsProdOutMax=[]  NTsProdOutMin=[]  NTsProdOutMax=[]  UintegralTsProdOutMin=[]  UintegralTsProdOutMax=[]  UngainTsProdOutMin=[]  UngainTsProdOutMax=[]  ClampingZeroOutDataTypeStr=Inherit: Inherit via back propagation  ClampingZeroOutMin=[]  ClampingZeroOutMax=[]  FilterDenConstantOutDataTypeStr=Inherit: Inherit via back propagation  FilterDenConstantOutMin=[]  FilterDenConstantOutMax=[]  PCopyOutDataTypeStr=Inherit: Inherit via back propagation  PCopyOutMin=[]  PCopyOutMax=[]  NCopyOutDataTypeStr=Inherit: Inherit via back propagation  NCopyOutMin=[]  NCopyOutMax=[]  IntegratorContinuousStateAttributes=''  IntegratorStateMustResolveToSignalObject=off  IntegratorRTWStateStorageClass=Auto  FilterContinuousStateAttributes=''  FilterStateMustResolveToSignalObject=off  FilterRTWStateStorageClass=Auto  ParallelPVariant=InternalParameters  IdealPVariant=Disabled  IVariant=InternalParameters  DVariant=InternalParameters  IntegratorVariant=Continuous  SatVariant=Enabled  AWVariant=Passthrough  PCopyVariant=Disabled  TRVariant=Disabled  FdbkBlocksVariant=Forward  IdealPFdbkVariant=Disabled  SatFdbkVariant=Disabled  DerivativeFilterVariant=ContFilter  NVariant=InternalParameters  NCopyVariant=Disabled  FilterICVariant=InternalICsFilter  IntegratorICVariant=InternalICs  ExternalResetVariant=Disabled  TRSumVariant=Passthrough  SumFdbkVariant=Disabled  SumVariant=Sum_PID  TsampFilterVariant=InternalTs  TsampNgainVariant=Passthrough  TsampIntegralVariant=Disabled_SignalSpec  ExternalSaturationOutDataTypeStr=Inherit: Same as second input  DerivativeSourceVariant=ErrorSignal
  PID Controller9 : slpidlib/PID Controller  Controller=PID  Form=Parallel  TimeDomain=Continuous-time  UseExternalTs=off  SampleTime=-1  IntegratorMethod=Forward Euler  FilterMethod=Forward Euler  ControllerParametersSource=internal  P=0.0886412010406481  I=0.0145723289748373  UseKiTs=off  D=0.129850691124493  UseExternalDerivativeSource=off  N=8.9831666478447  UseFilter=on  TunerSelectOption=Transfer Function Based (PID Tuner App)  InitialConditionSource=internal  InitialConditionForIntegrator=0  InitialConditionForFilter=0  DifferentiatorICPrevScaledInput=0  ExternalReset=none  TrackingMode=off  Kt=1  LimitOutput=on  SatLimitsSource=internal  UpperSaturationLimit=0.09  LowerSaturationLimit=-0.3  LinearizeAsGain=off  AntiWindupMode=clamping  Kb=1  LimitIntegrator=off  UpperIntegratorSaturationLimit=inf  LowerIntegratorSaturationLimit=-inf  POutMin=[]  POutMax=[]  IOutMin=[]  IOutMax=[]  DOutMin=[]  DOutMax=[]  NOutMin=[]  NOutMax=[]  SumOutMin=[]  SumOutMax=[]  SaturationOutMin=[]  SaturationOutMax=[]  PParamMin=[]  PParamMax=[]  IParamMin=[]  IParamMax=[]  DParamMin=[]  DParamMax=[]  NParamMin=[]  NParamMax=[]  KbParamMin=[]  KbParamMax=[]  KtParamMin=[]  KtParamMax=[]  KbOutMin=[]  KbOutMax=[]  KtOutMin=[]  KtOutMax=[]  IntegratorOutMin=[]  IntegratorOutMax=[]  FilterOutMin=[]  FilterOutMax=[]  SumI1OutMin=[]  SumI1OutMax=[]  SumI2OutMin=[]  SumI2OutMax=[]  SumI3OutMin=[]  SumI3OutMax=[]  SumI4OutMin=[]  SumI4OutMax=[]  SumDOutMin=[]  SumDOutMax=[]  DifferentiatorOutMin=[]  DifferentiatorOutMax=[]  FilterDiffOutCoefMin=[]  FilterDiffOutCoefMax=[]  ReciprocalOutMin=[]  ReciprocalOutMax=[]  SumDenOutMin=[]  SumDenOutMax=[]  SumNumOutMin=[]  SumNumOutMax=[]  DivideOutMin=[]  DivideOutMax=[]  UdiffTsProdOutMin=[]  UdiffTsProdOutMax=[]  NTsProdOutMin=[]  NTsProdOutMax=[]  UintegralTsProdOutMin=[]  UintegralTsProdOutMax=[]  UngainTsProdOutMin=[]  UngainTsProdOutMax=[]  ClampingZeroOutDataTypeStr=Inherit: Inherit via back propagation  ClampingZeroOutMin=[]  ClampingZeroOutMax=[]  FilterDenConstantOutDataTypeStr=Inherit: Inherit via back propagation  FilterDenConstantOutMin=[]  FilterDenConstantOutMax=[]  PCopyOutDataTypeStr=Inherit: Inherit via back propagation  PCopyOutMin=[]  PCopyOutMax=[]  NCopyOutDataTypeStr=Inherit: Inherit via back propagation  NCopyOutMin=[]  NCopyOutMax=[]  IntegratorContinuousStateAttributes=''  IntegratorStateMustResolveToSignalObject=off  IntegratorRTWStateStorageClass=Auto  FilterContinuousStateAttributes=''  FilterStateMustResolveToSignalObject=off  FilterRTWStateStorageClass=Auto  ParallelPVariant=InternalParameters  IdealPVariant=Disabled  IVariant=InternalParameters  DVariant=InternalParameters  IntegratorVariant=Continuous  SatVariant=Enabled  AWVariant=ContClampingParallel  PCopyVariant=Disabled  TRVariant=Disabled  FdbkBlocksVariant=Forward  IdealPFdbkVariant=Disabled  SatFdbkVariant=Disabled  DerivativeFilterVariant=ContFilter  NVariant=InternalParameters  NCopyVariant=Disabled  FilterICVariant=InternalICsFilter  IntegratorICVariant=InternalICs  ExternalResetVariant=Disabled  TRSumVariant=Passthrough  SumFdbkVariant=Disabled  SumVariant=Sum_PID  TsampFilterVariant=InternalTs  TsampNgainVariant=Passthrough  TsampIntegralVariant=Disabled_SignalSpec  ExternalSaturationOutDataTypeStr=Inherit: Same as second input  DerivativeSourceVariant=ErrorSignal
  Step demand for testing : Subsystem
  Step demand for testing1 : Subsystem
  Step demand for testing2 : Subsystem
  Subtract : Sum  Inputs=|-+
  Subtract1 : Sum  Inputs=|+-
  Subtract2 : Sum  Inputs=|+-
  Subtract3 : Sum  Inputs=|-+
  Subtract5 : Sum  Inputs=|+-
  Terminator : Terminator
  Terminator1 : Terminator
  Terminator2 : Terminator
  U : Outport
  wires:
  Mux/1 -> U/1
  h (z)/1 -> Step demand for testing/1(In1), Subtract1/1
  Subtract1/1 -> PID Controller9/1
  Subtract5/1 -> PID Controller1/1
  Va/1 -> Step demand for testing1/1(Va), Subtract5/1
  Subtract3/1 -> PID Controller10/1
  states/1 -> Get angular properties/2(In2)
  Get angular properties/1(Flight Trajectory (gamma)) -> Subtract/2
  Get angular properties/2(Pitch rate (q)) -> Subtract3/2
  alpha/1 -> Get angular properties/1(alpha)
  Get angular properties/3(ub) -> Terminator/1
  PID Controller1/1 -> Mux/4
  Get angular properties/6(Course Angle) -> Step demand for testing2/1(Va), Subtract2/1
  Get angular properties/4(Roll Rate (p)) -> Terminator1/1
  PID Controller9/1 -> Subtract/1
  PID Controller10/1 -> Mux/1
  Get angular properties/5(Yaw Rate (r)) -> Terminator2/1
  Subtract2/1 -> PID Controller7/1, PID Controller2/1
  PID Controller7/1 -> Mux/2
  PID Controller2/1 -> Mux/3
  PID Controller4/1 -> Subtract3/1
  Constant1/1 -> Subtract5/2
  Step demand for testing/1(Out1) -> Subtract1/2
  Subtract/1 -> PID Controller4/1
